simulink model "multipleFSM_demo_tests"  (R2019b)
settings: Solver=FixedStepDiscrete  StartTime=0  StopTime=100  RelTol=1e-3
libraries: simulink x2
settings Model: Creator=cyarp  LastModifiedBy=cyarp

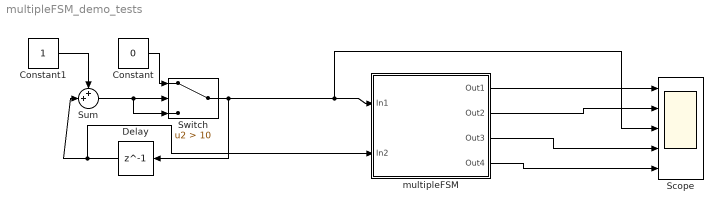
== system multipleFSM_demo_tests ==
  Constant : Constant  Value=0  OutDataTypeStr=single
  Constant1 : Constant  OutDataTypeStr=single
  Delay : Delay  DelayLength=1  SampleTime=4
  Scope : Scope  NumInputPorts=5
  Sum : Sum  Inputs=++|
  Switch : Switch  Criteria=u2 > Threshold  Threshold=10
  multipleFSM : Subsystem
  wires:
  Delay/1 -> multipleFSM/2(In2), Sum/2
  Switch/1 -> Delay/1, Scope/3, multipleFSM/1(In1)
  Sum/1 -> Switch/2, Switch/3
  Constant/1 -> Switch/1
  Constant1/1 -> Sum/1
  multipleFSM/1(Out1) -> Scope/1
  multipleFSM/2(Out2) -> Scope/2
  multipleFSM/3(Out3) -> Scope/4
  multipleFSM/4(Out4) -> Scope/5

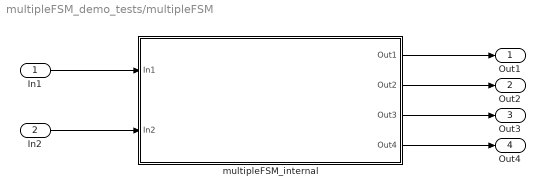
== system multipleFSM_demo_tests/multipleFSM ==
  In1 : Inport
  In2 : Inport  Port=2
  multipleFSM_internal : Subsystem
  Out1 : Outport
  Out2 : Outport  Port=2
  Out3 : Outport  Port=3
  Out4 : Outport  Port=4
  wires:
  In1/1 -> multipleFSM_internal/1(In1)
  In2/1 -> multipleFSM_internal/2(In2)
  multipleFSM_internal/1(Out1) -> Out1/1
  multipleFSM_internal/2(Out2) -> Out2/1
  multipleFSM_internal/4(Out4) -> Out4/1
  multipleFSM_internal/3(Out3) -> Out3/1

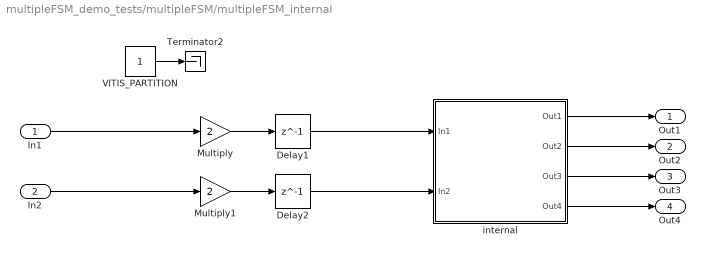
== system multipleFSM_demo_tests/multipleFSM/multipleFSM_internal ==
  In1 : Inport
  In2 : Inport  Port=2
  Delay1 : Delay  DelayLength=1
  Delay2 : Delay  DelayLength=1
  Multiply : Gain  Gain=2
  Multiply1 : Gain  Gain=2
  Terminator2 : Terminator
  VITIS_PARTITION : Constant
  internal : Subsystem
  Out1 : Outport
  Out2 : Outport  Port=2
  Out3 : Outport  Port=3
  Out4 : Outport  Port=4
  wires:
  In1/1 -> Multiply/1
  In2/1 -> Multiply1/1
  Multiply1/1 -> Delay2/1
  Delay1/1 -> internal/1(In1)
  internal/2(Out2) -> Out2/1
  Multiply/1 -> Delay1/1
  Delay2/1 -> internal/2(In2)
  internal/1(Out1) -> Out1/1
  VITIS_PARTITION/1 -> Terminator2/1
  internal/3(Out3) -> Out3/1
  internal/4(Out4) -> Out4/1

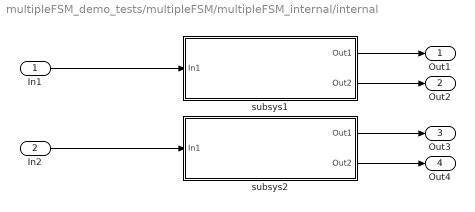
== system multipleFSM_demo_tests/multipleFSM/multipleFSM_internal/internal ==
  In1 : Inport
  In2 : Inport  Port=2
  subsys1 : Subsystem
  subsys2 : Subsystem
  Out1 : Outport
  Out2 : Outport  Port=2
  Out3 : Outport  Port=3
  Out4 : Outport  Port=4
  wires:
  In1/1 -> subsys1/1(In1)
  In2/1 -> subsys2/1(In1)
  subsys1/1(Out1) -> Out1/1
  subsys1/2(Out2) -> Out2/1
  subsys2/1(Out1) -> Out3/1
  subsys2/2(Out2) -> Out4/1

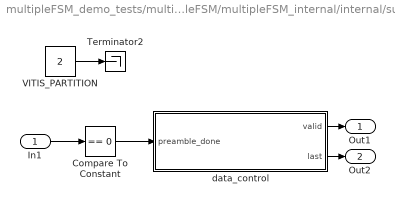
== system multipleFSM_demo_tests/multipleFSM/multipleFSM_internal/internal/subsys1 ==
  In1 : Inport
  Compare To Constant : simulink/Logic and Bit Operations/Compare To Constant  relop===  const=0  OutDataTypeStr=boolean
  Terminator2 : Terminator
  VITIS_PARTITION : Constant  Value=2
  data_control : Stateflow chart  AncestorBlock=<binary blob, 156 chars, not shown>  TreatAsAtomicUnit=on
  Out1 : Outport
  Out2 : Outport  Port=2
  wires:
  data_control/1(valid) -> Out1/1
  In1/1 -> Compare To Constant/1
  data_control/2(last) -> Out2/1
  Compare To Constant/1 -> data_control/1(preamble_done)
  VITIS_PARTITION/1 -> Terminator2/1

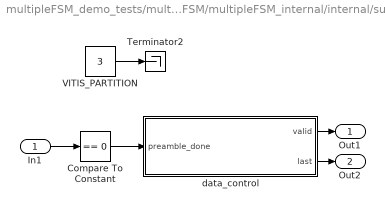
== system multipleFSM_demo_tests/multipleFSM/multipleFSM_internal/internal/subsys2 ==
  In1 : Inport
  Compare To Constant : simulink/Logic and Bit Operations/Compare To Constant  relop===  const=0  OutDataTypeStr=boolean
  Terminator2 : Terminator
  VITIS_PARTITION : Constant  Value=3
  data_control : Stateflow chart  AncestorBlock=<binary blob, 156 chars, not shown>  TreatAsAtomicUnit=on
  Out1 : Outport
  Out2 : Outport  Port=2
  wires:
  data_control/1(valid) -> Out1/1
  In1/1 -> Compare To Constant/1
  data_control/2(last) -> Out2/1
  Compare To Constant/1 -> data_control/1(preamble_done)
  VITIS_PARTITION/1 -> Terminator2/1

== stateflow chart multipleFSM_demo_tests/multipleFSM/multipleFSM_internal/internal/subsys2/data_control ==
  settings: executeAtInitialization=1
  state Data
    entry:
    valid = true;
    last = false;
    dataCount = dataCount + int32(1);
  state LastSym
    entry:
    valid = true;
    last = true;
    dataCount = dataCount + int32(1);
  state Waiting
    entry:
    valid = false;
    last = false;
    startCount = int32(0);
    dataCount = int32(0);
    waitCount = int32(0);
  state DummyInit
    entry:
    valid = false;
    last = false;
    startCount = int32(0);
    dataCount = int32(0);
    waitCount = int32(0);
  Data -> Data [order 2]
  (default) -> DummyInit
  Waiting -> Data : [preamble_done == true]
  DummyInit -> Waiting
  LastSym -> Waiting
  Data -> LastSym [order 1] : [dataCount >= dataLenSymbols-1]
  data: preamble_done input boolean; valid output boolean; startCount local int32; dataCount local int32; buffer local boolean size=8; guardInt local int32 =int32(10); guardTol local int32 =int32(10); waitCount local int32 =int32(10); wordLen local int32 =int32(10); dataLenSymbols local int32 =int32(10); last output boolean

== stateflow chart multipleFSM_demo_tests/multipleFSM/multipleFSM_internal/internal/subsys1/data_control ==
  settings: executeAtInitialization=1
  state Data
    entry:
    valid = true;
    last = false;
    dataCount = dataCount + int32(1);
  state LastSym
    entry:
    valid = true;
    last = true;
    dataCount = dataCount + int32(1);
  state Waiting
    entry:
    valid = false;
    last = false;
    startCount = int32(0);
    dataCount = int32(0);
    waitCount = int32(0);
  state DummyInit
    entry:
    valid = false;
    last = false;
    startCount = int32(0);
    dataCount = int32(0);
    waitCount = int32(0);
  Data -> Data [order 2]
  (default) -> DummyInit
  Waiting -> Data : [preamble_done == true]
  DummyInit -> Waiting
  LastSym -> Waiting
  Data -> LastSym [order 1] : [dataCount >= dataLenSymbols-1]
  data: preamble_done input boolean; valid output boolean; startCount local int32; dataCount local int32; buffer local boolean size=8; guardInt local int32 =int32(10); guardTol local int32 =int32(10); waitCount local int32 =int32(10); wordLen local int32 =int32(10); dataLenSymbols local int32 =int32(10); last output boolean
